simulink model "mod_02"  (R2017b)
settings: Solver=VariableStepAuto  StartTime=0.0  StopTime=20.0  RelTol=1e-3
settings Model: Creator=Manu  LastModifiedBy=Manu

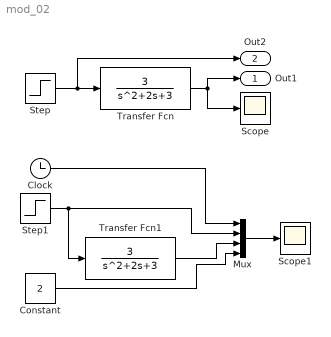
== system mod_02 ==
  Clock : Clock
  Constant : Constant  Value=2
  Mux : Mux
  Scope : Scope
  Scope1 : Scope
  Step : Step  SampleTime=0
  Step1 : Step  SampleTime=0
  Transfer Fcn : TransferFcn  Numerator=[3]  Denominator=[1 2 3]
  Transfer Fcn1 : TransferFcn  Numerator=[3]  Denominator=[1 2 3]
  Out1 : Outport
  Out2 : Outport  Port=2
  wires:
  Step/1 -> Out2/1, Transfer Fcn/1
  Transfer Fcn/1 -> Scope/1, Out1/1
  Step1/1 -> Transfer Fcn1/1, Mux/2
  Clock/1 -> Mux/1
  Constant/1 -> Mux/4
  Transfer Fcn1/1 -> Mux/3
  Mux/1 -> Scope1/1
